simulink model "Devcon"  (R2022a)
settings: Solver=VariableStepAuto  StartTime=0.0  StopTime=20  RelTol=1e-3
settings Model: Creator=jaybee  LastModifiedBy=jaybee

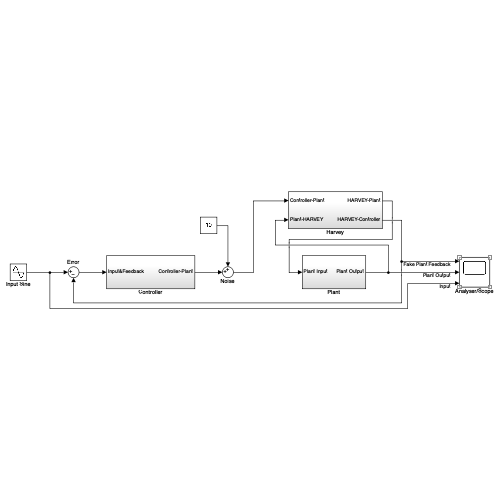
[thumbnail: Simulink's stored preview of the top-level diagram]
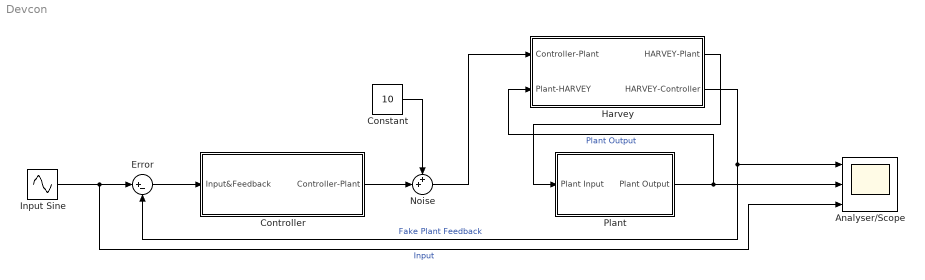
== system Devcon ==
  Analyser/Scope : Scope  NumInputPorts=3
  Constant : Constant  Value=10
  Controller : Subsystem
  Error : Sum  Inputs=|+-
  Harvey : Subsystem
  Input Sine : Sin  Frequency=5  SampleTime=0
  Noise : Sum  Inputs=++|
  Plant : Subsystem
  wires:
  Error/1 -> Controller/1(Input&Feedback)
  Controller/1(Controller-Plant) -> Noise/2
  Input Sine/1 -> Analyser/Scope/3, Error/1  "Input"
  Constant/1 -> Noise/1
  Noise/1 -> Harvey/1(Controller-Plant)
  Harvey/2(HARVEY-Controller) -> Analyser/Scope/1, Error/2  "Fake Plant Feedback"
  Plant/1(Plant Output) -> Harvey/2(Plant-HARVEY), Analyser/Scope/2  "Plant Output"
  Harvey/1(HARVEY-Plant) -> Plant/1(Plant Input)

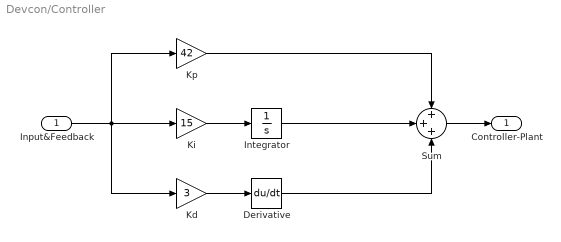
== system Devcon/Controller ==
  Input&Feedback : Inport
  Derivative : Derivative
  Integrator : Integrator
  Kd : Gain  Gain=3
  Ki : Gain  Gain=15
  Kp : Gain  Gain=42
  Sum : Sum  Inputs=+++
  Controller-Plant : Outport
  wires:
  Sum/1 -> Controller-Plant/1
  Kd/1 -> Derivative/1
  Ki/1 -> Integrator/1
  Input&Feedback/1 -> Ki/1, Kd/1, Kp/1
  Kp/1 -> Sum/1
  Integrator/1 -> Sum/2
  Derivative/1 -> Sum/3

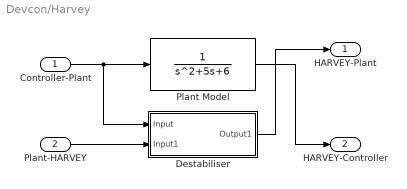
== system Devcon/Harvey ==
  Controller-Plant : Inport
  Plant-HARVEY : Inport  Port=2
  " Plant Model" : TransferFcn  Denominator=[1 5 6]
  Destabiliser : Subsystem
  HARVEY-Plant : Outport
  HARVEY-Controller : Outport  Port=2
  wires:
  Controller-Plant/1 -> Destabiliser/1(Input), " Plant Model"/1
  " Plant Model"/1 -> HARVEY-Controller/1
  Destabiliser/1(Output1) -> HARVEY-Plant/1
  Plant-HARVEY/1 -> Destabiliser/2(Input1)

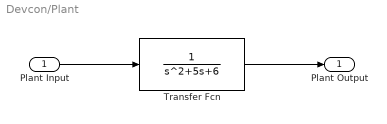
== system Devcon/Plant ==
  Plant Input : Inport
  Transfer Fcn : TransferFcn  Denominator=[1 5 6]
  Plant Output : Outport
  wires:
  Plant Input/1 -> Transfer Fcn/1
  Transfer Fcn/1 -> Plant Output/1

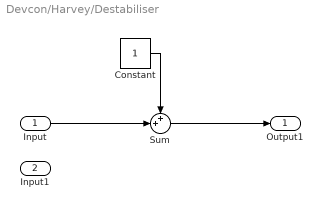
== system Devcon/Harvey/Destabiliser ==
  Input : Inport
  Input1 : Inport  Port=2
  Constant : Constant
  Sum : Sum  Inputs=++|
  Output1 : Outport
  wires:
  Sum/1 -> Output1/1
  Constant/1 -> Sum/1
  Input/1 -> Sum/2
